simulink model "class_wala"  (R2021a)
settings: Solver=VariableStepAuto  StartTime=0.0  StopTime=10  RelTol=1e-3
settings Model: Creator=Abhishek Agarwal  LastModifiedBy=Abhishek Agarwal

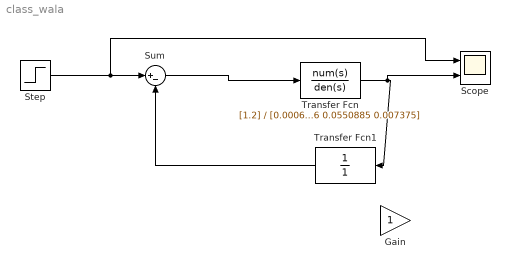
== system class_wala ==
  Gain : Gain
  Scope : Scope  NumInputPorts=2
  Step : Step  Time=0.5  Before=500  After=1000  SampleTime=0
  Sum : Sum  Inputs=|+-
  Transfer Fcn : TransferFcn  Numerator=[1.2]  Denominator=[0.00066 0.0550885 0.007375]
  Transfer Fcn1 : TransferFcn  Denominator=[1]
  wires:
  Sum/1 -> Transfer Fcn/1
  Transfer Fcn1/1 -> Sum/2
  Transfer Fcn/1 -> Scope/2, Transfer Fcn1/1
  Step/1 -> Scope/1, Sum/1
